simulink model "Control_Scheme_Joint_PID_Simulink"  (R2021a)
settings: Solver=FixedStepAuto  StartTime=0.0  StopTime=8  FixedStep=0.001  RelTol=1e-20
libraries: simulink x10, pid_lib x8
(part 2 of 2)

== matlab function Control_Scheme_Joint_PID_Simulink/MATLAB Function5 ==
  data: tao_in input; q output; t_in input; q_1 input; q_dot_1 input; q_dot output
function [q,q_dot] = SCDPR_Func(tao_in,t_in,q_1,q_dot_1)
% 主要求解电机的动力学方程，通过给定电机转矩以及索力信息，得到电机的角度以及角速度
%   此处显示详细说明

% global tao;
tao=tao_in;
% global tt;
tt=t_in;
% global Im;
Im=[0.1 0.1 0.1 0.1 0.1 0.1 0.1 0.1 0.1]';
% global Fv;
Fv=[1 1 1 1 1 1 1 1]';
% global Fs;
Fs=[1 1 1 1 1 1 1 1]';
% global R;
R=[0.0225 0.0225 0.0225 0.0225 0.0225 0.0225 0.0225 0.0225]';

T=0.001;
% T=0.01;

q=zeros(8,1);
q_dot=zeros(8,1);


% 第1个微分方程
Y11=q_1(1);
Y21=q_dot_1(1);
% 解微分方程
[t,q1] = ode45(@vdp1,[0 T],[Y11; Y21],[],tao,tt,Im,Fv,Fs,R);
q(1)=q1(end,1);
q_dot(1)=q1(end,2);

% 第2个微分方程
Y12=q_1(2);
Y22=q_dot_1(2);
% 解微分方程
[t,q2] = ode45(@vdp2,[0 T],[Y12; Y22],[],tao,tt,Im,Fv,Fs,R);
q(2)=q2(end,1);
q_dot(2)=q2(end,2);

% 第3个微分方程
Y13=q_1(3);
Y23=q_dot_1(3);
% 解微分方程
[t,q3] = ode45(@vdp3,[0 T],[Y13; Y23],[],tao,tt,Im,Fv,Fs,R);
q(3)=q3(end,1);
q_dot(3)=q3(end,2);

% 第4个微分方程
Y14=q_1(4);
Y24=q_dot_1(4);
% 解微分方程
[t,q4] = ode45(@vdp4,[0 T],[Y14; Y24],[],tao,tt,Im,Fv,Fs,R);
q(4)=q4(end,1);
q_dot(4)=q4(end,2);

% 第5个微分方程
Y15=q_1(5);
Y25=q_dot_1(5);
% 解微分方程
[t,q5] = ode45(@vdp5,[0 T],[Y15; Y25],[],tao,tt,Im,Fv,Fs,R);
q(5)=q5(end,1);
q_dot(5)=q5(end,2);

% 第6个微分方程
Y16=q_1(6);
Y26=q_dot_1(6);
% 解微分方程
[t,q6] = ode45(@vdp6,[0 T],[Y16; Y26],[],tao,tt,Im,Fv,Fs,R);
q(6)=q6(end,1);
q_dot(6)=q6(end,2);

% 第7个微分方程
Y17=q_1(7);
Y27=q_dot_1(7);
% 解微分方程
[t,q7] = ode45(@vdp7,[0 T],[Y17; Y27],[],tao,tt,Im,Fv,Fs,R);
q(7)=q7(end,1);
q_dot(7)=q7(end,2);

% 第8个微分方程
Y18=q_1(8);
Y28=q_dot_1(8);
% 解微分方程
[t,q8] = ode45(@vdp8,[0 T],[Y18; Y28],[],tao,tt,Im,Fv,Fs,R);
q(8)=q8(end,1);
q_dot(8)=q8(end,2);

function dydt1 = vdp1(t,y,tao,tt,Im,Fv,Fs,R)
%     global tao;
%     global tt;
%     global Im;
%     global Fv;
%     global Fs;
%     global R;
    
    tao1=tao(1);
    tt1=tt(1);
    Im1=Im(1);
    Fv1=Fv(1);
    Fs1=Fs(1);
    R1=R(1);

    p = y(1);
    dp = y(2);
% 	ddp = -Im_inv*Fv*dp-Im_inv*Fs*sign(dp)+Im_inv*tao-Im_inv*R*tt;
    ddp = -Fv1/Im1*dp-Fs1/Im1*sign(dp)+tao1/Im1-R1/Im1*tt1;
    dydt1 = [dp; ddp];
end

function dydt2 = vdp2(t,y,tao,tt,Im,Fv,Fs,R)
%     global tao;
%     global tt;
%     global Im;
%     global Fv;
%     global Fs;
%     global R;
    
    tao2=tao(2);
    tt2=tt(2);
    Im2=Im(2);
    Fv2=Fv(2);
    Fs2=Fs(2);
    R2=R(2);

    p = y(1);
    dp = y(2);
% 	ddp = -Im_inv*Fv*dp-Im_inv*Fs*sign(dp)+Im_inv*tao-Im_inv*R*tt;
    ddp = -Fv2/Im2*dp-Fs2/Im2*sign(dp)+tao2/Im2-R2/Im2*tt2;
    dydt2 = [dp; ddp];
end

function dydt3 = vdp3(t,y,tao,tt,Im,Fv,Fs,R)
%     global tao;
%     global tt;
%     global Im;
%     global Fv;
%     global Fs;
%     global R;
    
    tao3=tao(3);
    tt3=tt(3);
    Im3=Im(3);
    Fv3=Fv(3);
    Fs3=Fs(3);
    R3=R(3);

    p = y(1);
    dp = y(2);
% 	ddp = -Im_inv*Fv*dp-Im_inv*Fs*sign(dp)+Im_inv*tao-Im_inv*R*tt;
    ddp = -Fv3/Im3*dp-Fs3/Im3*sign(dp)+tao3/Im3-R3/Im3*tt3;
    dydt3 = [dp; ddp];
end

function dydt4 = vdp4(t,y,tao,tt,Im,Fv,Fs,R)
%     global tao;
%     global tt;
%     global Im;
%     global Fv;
%     global Fs;
%     global R;
    
    tao4=tao(4);
    tt4=tt(4);
    Im4=Im(4);
    Fv4=Fv(4);
    Fs4=Fs(4);
    R4=R(4);

    p = y(1);
    dp = y(2);
% 	ddp = -Im_inv*Fv*dp-Im_inv*Fs*sign(dp)+Im_inv*tao-Im_inv*R*tt;
    ddp = -Fv4/Im4*dp-Fs4/Im4*sign(dp)+tao4/Im4-R4/Im4*tt4;
    dydt4 = [dp; ddp];
end

function dydt5 = vdp5(t,y,tao,tt,Im,Fv,Fs,R)
%     global tao;
%     global tt;
%     global Im;
%     global Fv;
%     global Fs;
%     global R;
    
    tao5=tao(5);
    tt5=tt(5);
    Im5=Im(5);
    Fv5=Fv(5);
    Fs5=Fs(5);
    R5=R(5);

    p = y(1);
    dp = y(2);
% 	ddp = -Im_inv*Fv*dp-Im_inv*Fs*sign(dp)+Im_inv*tao-Im_inv*R*tt;
    ddp = -Fv5/Im5*dp-Fs5/Im5*sign(dp)+tao5/Im5-R5/Im5*tt5;
    dydt5 = [dp; ddp];
end

function dydt6 = vdp6(t,y,tao,tt,Im,Fv,Fs,R)
%     global tao;
%     global tt;
%     global Im;
%     global Fv;
%     global Fs;
%     global R;
    
    tao6=tao(6);
    tt6=tt(6);
    Im6=Im(6);
    Fv6=Fv(6);
    Fs6=Fs(6);
    R6=R(6);

    p = y(1);
    dp = y(2);
% 	ddp = -Im_inv*Fv*dp-Im_inv*Fs*sign(dp)+Im_inv*tao-Im_inv*R*tt;
    ddp = -Fv6/Im6*dp-Fs6/Im6*sign(dp)+tao6/Im6-R6/Im6*tt6;
    dydt6 = [dp; ddp];
end


function dydt7 = vdp7(t,y,tao,tt,Im,Fv,Fs,R)
%     global tao;
%     global tt;
%     global Im;
%     global Fv;
%     global Fs;
%     global R;
    
    tao7=tao(7);
    tt7=tt(7);
    Im7=Im(7);
    Fv7=Fv(7);
    Fs7=Fs(7);
    R7=R(7);

    p = y(1);
    dp = y(2);
% 	ddp = -Im_inv*Fv*dp-Im_inv*Fs*sign(dp)+Im_inv*tao-Im_inv*R*tt;
    ddp = -Fv7/Im7*dp-Fs7/Im7*sign(dp)+tao7/Im7-R7/Im7*tt7;
    dydt7 = [dp; ddp];
end

function dydt8 = vdp8(t,y,tao,tt,Im,Fv,Fs,R)
%     global tao;
%     global tt;
%     global Im;
%     global Fv;
%     global Fs;
%     global R;
    
    tao8=tao(8);
    tt8=tt(8);
    Im8=Im(8);
    Fv8=Fv(8);
    Fs8=Fs(8);
    R8=R(8);

    p = y(1);
    dp = y(2);
% 	ddp = -Im_inv*Fv*dp-Im_inv*Fs*sign(dp)+Im_inv*tao-Im_inv*R*tt;
    ddp = -Fv8/Im8*dp-Fs8/Im8*sign(dp)+tao8/Im8-R8/Im8*tt8;
    dydt8 = [dp; ddp];
end
end

== matlab function Control_Scheme_Joint_PID_Simulink/MATLAB Function6 ==
  data: t input; q_1 output size=[8,1] [8..8]; qd input; qd_dot input; q input; q_dot input; q_dot_1 output
function [q_1,q_dot_1] = Select_q_and_q_dot(t,qd,qd_dot,q,q_dot)

q_1=zeros(8,1);
q_dot_1=zeros(8,1);

if t<=3e-3
    q_1=qd;
    q_dot_1=qd_dot;
else
    q_1=q;
    q_dot_1=q_dot;
%     q_dot_1=qd_dot;
end

end

== matlab function Control_Scheme_Joint_PID_Simulink/MATLAB Function7 ==
  data: p input; t output; theta input; we input; bool output
function [t,bool] = Tension_Distribution_Func(p,theta,we)
% 求解索力分布的函数
% 输入：p 动平台位置 3*1
%      theta 动平台坐标系XYZ欧拉角 3*1
%      we 动平台受到的wrench 6*1(包含本身质量)
% 输出：t 绳索的张力的大小 8*1

g=9.81; %重力加速度
theta=theta';
x=theta(1);
y=theta(2);
z=theta(3);
Rxyz=Theta2RotationMatrix_Func(x,y,z);
f=we;
%% CoGiRo的参数 8绳索6自由度的CDPRs
% ai的定义
a1=[-7.5 -5.5 6]';
a2=[-7.5 -5.5 6]';
a3=[-7.5 5.5 6]';
a4=[-7.5 5.5 6]';
a5=[7.5 5.5 6]';
a6=[7.5 5.5 6]';
a7=[7.5 -5.5 6]';
a8=[7.5 -5.5 6]';
% bi的定义
b1=Rxyz*[0.5 -0.5 0]';
b2=Rxyz*[-0.5 0.5 1]';
b3=Rxyz*[-0.5 -0.5 0]';
b4=Rxyz*[0.5 0.5 1]';
b5=Rxyz*[-0.5 0.5 0]';
b6=Rxyz*[0.5 -0.5 1]';
b7=Rxyz*[0.5 0.5 0]';
b8=Rxyz*[-0.5 -0.5 1]';
% 绳索张力的上下限
tM=1000;
tm=10;
%% li=ai-bi-p,然后归一化li得到si=li/norm(li)
% li=ai-bi-p
l1=a1-b1-p;
l2=a2-b2-p;
l3=a3-b3-p;
l4=a4-b4-p;
l5=a5-b5-p;
l6=a6-b6-p;
l7=a7-b7-p;
l8=a8-b8-p;
% for i=1:8
%     expr=['l',num2str(i),'=a',num2str(i),'-b',num2str(i),'-p;'];
%     eval(expr);
% end
% si=li/norm(li)
s1=l1/norm(l1);
s2=l2/norm(l2);
s3=l3/norm(l3);
s4=l4/norm(l4);
s5=l5/norm(l5);
s6=l6/norm(l6);
s7=l7/norm(l7);
s8=l8/norm(l8);

% for i=1:8
%     expr=['s',num2str(i),'=l',num2str(i),'./norm(l',num2str(i),');'];
%     eval(expr);
% end

%% 构建W矩阵
% wi=[si;cross(bi,si)]
w1=[s1;cross(b1,s1)];
w2=[s2;cross(b2,s2)];
w3=[s3;cross(b3,s3)];
w4=[s4;cross(b4,s4)];
w5=[s5;cross(b5,s5)];
w6=[s6;cross(b6,s6)];
w7=[s7;cross(b7,s7)];
w8=[s8;cross(b8,s8)];
W=[w1 w2 w3 w4 w5 w6 w7 w8];

W_plus=pinv(W);
N=null(W);
tp=W_plus*f;

tm_vec=[tm;tm;tm;tm;tm;tm;tm;tm;];
tM_vec=[tM;tM;tM;tM;tM;tM;tM;tM;];

% line_select=[];
% langda_select=[];

find=0;
k_vector_all=[1;2;3;4;5;6;7;8];

%% 寻找第一个顶点vinit
i=1;
j=2;
bi=tm;
bj=tm;
bk_1=0;
bk_2=0;
ni=N(i,:);
nj=N(j,:);
tpi=tp(i,:);
tpj=tp(j,:);
A=[ni;nj];
b=[bi-tpi;bj-tpj];
langda=A\b; %2*1向量
vij=langda;

% line_select=[line_select;j];
% line_select=[line_select;i];
line_select=[i];

lk_1=i;
lk_2=j;

% line_find=[];
% line_find=[line_find;1];
% line_find=[line_find;2];
line_find=[i;j];

for i=3:8
    ni_2=N(i,:);
    tpi_2=tp(i,:);
    if ni_2*langda>=tm-tpi_2 & ni_2*langda<=tM-tpi_2
        line_find=[line_find;i];
    end
    
end

langda_select=[vij];


k_vector=setdiff(k_vector_all,line_select);

%% 循环找下一个节点，直到找到vk==vf
vk=[1e30;1e30];
% alpah_v=[1e30;1e30];
alpah_v=[1e30];
vk_1=vij;
nk_1=ni;
nk_2=nj;
nk_1_vertical=null(nk_1)';
nk_2_vertical=null(nk_2)';
l=0;
bk=0;
tpk=0;
count=0;
find2=0;
vf=vij;
vf_count=count+1;
nk_1_vertical_final=[0 0];
while(1)
%     alpah_k=[1e30;1e30];
    alpah_k=[1e30];
    count=count+1;
    find2=0;
    nk_1_vertical_final=[0 0];
    for i=1:length(k_vector)
        k=k_vector(i);
        nk=N(k,:);
        tpk=tp(k,:);
        
        % 考虑bj=tm情况
        if bk_2==0           
            nk_1_vertical_1=[nk_1(2) -nk_1(1)];
            nk_1_vertical_2=[-nk_1(2) nk_1(1)];
%             nk_1_vertical_1=[-nk_1(2) nk_1(1)];
%             nk_1_vertical_2=[nk_1(2) -nk_1(1)];
            if nk_2*nk_1_vertical_1'>=0
                nk_1_vertical=nk_1_vertical_1;
            else
                nk_1_vertical=nk_1_vertical_2;
            end           
            
            if nk*nk_1_vertical'>0
                if k==lk_2
                    if nk*vk_1<=tm-tpk
                        alpah_k=(tM-tpk-nk*vk_1)/(nk*nk_1_vertical');
                        bk_tmp=1;
                    elseif nk*vk_1>tm-tpk & nk*vk_1<=tM-tpk
                        alpah_k=(tM-tpk-nk*vk_1)/(nk*nk_1_vertical');
                        bk_tmp=1;
                    else
                        bk_tmp=0;
                    end
%                     if nk*vk_1>tm-tpk & nk*vk_1<=tM-tpk
%                         alpah_k=(tM-tpk-nk*vk_1)/(nk*nk_1_vertical');
%                         bk_tmp=1;
%                     end
                else
                    if nk*vk_1<=tm-tpk
                        alpah_k=(tm-tpk-nk*vk_1)/(nk*nk_1_vertical');
                        bk_tmp=0;
                    elseif nk*vk_1>tm-tpk & nk*vk_1<=tM-tpk
                        alpah_k=(tM-tpk-nk*vk_1)/(nk*nk_1_vertical');
                        bk_tmp=1;
                    else
                        bk_tmp=0;
                    end
%                     if nk*vk_1>tm-tpk & nk*vk_1<=tM-tpk
%                         alpah_k=(tM-tpk-nk*vk_1)/(nk*nk_1_vertical');
%                         bk_tmp=1;
%                     end
                end
                if (alpah_k<alpah_v) & alpah_k>=1e-6
                    alpah_v=alpah_k;
                    l=k;
                    find2=1;
                    nk_1_vertical_final=nk_1_vertical;
                    bk=bk_tmp;
                else
                    
                end
            end

            if nk*nk_1_vertical'<0
                if k==lk_2
                    if nk*vk_1>=tM-tpk
                        alpah_k=(tm-tpk-nk*vk_1)/(nk*nk_1_vertical');
                        bk_tmp=0;
                    elseif nk*vk_1>=tm-tpk & nk*vk_1<tM-tpk
                        alpah_k=(tm-tpk-nk*vk_1)/(nk*nk_1_vertical');
                        bk_tmp=0;
                    else
                        bk_tmp=0;
                    end
%                     if nk*vk_1>=tm-tpk & nk*vk_1<tM-tpk
%                         alpah_k=(tm-tpk-nk*vk_1)/(nk*nk_1_vertical');
%                         bk_tmp=0;
%                     end
                else
                    if nk*vk_1>=tM-tpk
                        alpah_k=(tM-tpk-nk*vk_1)/(nk*nk_1_vertical');
                        bk_tmp=1;
                    elseif nk*vk_1>=tm-tpk & nk*vk_1<tM-tpk
                        alpah_k=(tm-tpk-nk*vk_1)/(nk*nk_1_vertical');
                        bk_tmp=0;
                    else
                        bk_tmp=0;
                    end
%                     if nk*vk_1>=tm-tpk & nk*vk_1<tM-tpk
%                         alpah_k=(tm-tpk-nk*vk_1)/(nk*nk_1_vertical');
%                         bk_tmp=0;
%                     end
                end
                if (alpah_k<alpah_v) & alpah_k>=1e-6
                    alpah_v=alpah_k;
                    l=k;
                    find2=1;
                    nk_1_vertical_final=nk_1_vertical;
                    bk=bk_tmp;
                else
                    
                end
            end
        
        % 考虑bk=tM的情况
        elseif bk_2==1
            nk_1_vertical_1=[nk_1(2) -nk_1(1)];
            nk_1_vertical_2=[-nk_1(2) nk_1(1)];
%             nk_1_vertical_1=[-nk_1(2) nk_1(1)];
%             nk_1_vertical_2=[nk_1(2) -nk_1(1)];
            if nk_2*nk_1_vertical_1'<=0
                nk_1_vertical=nk_1_vertical_1;
            else
                nk_1_vertical=nk_1_vertical_2;
            end

            if nk*nk_1_vertical'>0
                if k==lk_2
                    if nk*vk_1<=tm-tpk
                        alpah_k=(tM-tpk-nk*vk_1)/(nk*nk_1_vertical');
                        bk_tmp=1;
                    elseif nk*vk_1>tm-tpk & nk*vk_1<=tM-tpk
                        alpah_k=(tM-tpk-nk*vk_1)/(nk*nk_1_vertical');
                        bk_tmp=1;
                    else
                        bk_tmp=0;
                    end
%                     if nk*vk_1>tm-tpk & nk*vk_1<=tM-tpk
%                         alpah_k=(tM-tpk-nk*vk_1)/(nk*nk_1_vertical');
%                         bk_tmp=1;
%                     end
                else
                    if nk*vk_1<=tm-tpk
                        alpah_k=(tm-tpk-nk*vk_1)/(nk*nk_1_vertical');
                        bk_tmp=0;
                    elseif nk*vk_1>tm-tpk & nk*vk_1<=tM-tpk
                        alpah_k=(tM-tpk-nk*vk_1)/(nk*nk_1_vertical');
                        bk_tmp=1;
                    else
                        bk_tmp=0;
                    end
%                     if nk*vk_1>tm-tpk & nk*vk_1<=tM-tpk
%                         alpah_k=(tM-tpk-nk*vk_1)/(nk*nk_1_vertical');
%                         bk_tmp=1;
%                     end
                end
                if (alpah_k<alpah_v) & alpah_k>=1e-6
                    alpah_v=alpah_k;
                    l=k;
                    find2=1;
                    nk_1_vertical_final=nk_1_vertical;
                    bk=bk_tmp;
                else
                    
                end
            end

            if nk*nk_1_vertical'<0
                if k==lk_2
                    if nk*vk_1>=tM-tpk
                        alpah_k=(tm-tpk-nk*vk_1)/(nk*nk_1_vertical');
                        bk_tmp=0;
                    elseif nk*vk_1>=tm-tpk & nk*vk_1<tM-tpk
                        alpah_k=(tm-tpk-nk*vk_1)/(nk*nk_1_vertical');
                        bk_tmp=0;
                    else
                        bk_tmp=0;
                    end
%                     if nk*vk_1>=tm-tpk & nk*vk_1<tM-tpk
%                         alpah_k=(tm-tpk-nk*vk_1)/(nk*nk_1_vertical');
%                         bk_tmp=0;
%                     end
                else
                    if nk*vk_1>=tM-tpk
                        alpah_k=(tM-tpk-nk*vk_1)/(nk*nk_1_vertical');
                        bk_tmp=1;
                    elseif nk*vk_1>=tm-tpk & nk*vk_1<tM-tpk
                        alpah_k=(tm-tpk-nk*vk_1)/(nk*nk_1_vertical');
                        bk_tmp=0;
                    else
                        bk_tmp=0;
                    end
%                     if nk*vk_1>=tm-tpk & nk*vk_1<tM-tpk
%                         alpah_k=(tm-tpk-nk*vk_1)/(nk*nk_1_vertical');
%                         bk_tmp=0;
%                     end
                end
                if (alpah_k<alpah_v) & alpah_k>=1e-6
                    alpah_v=alpah_k;
                    l=k;
                    find2=1;
                    nk_1_vertical_final=nk_1_vertical;
                    bk=bk_tmp;
                else
                    
                end
            end
        else
            find2=0;
        end
    end
    if find2==0 || count>1000
        t=[0 0 0 0 0 0 0 0]';
        bool=0;
%         disp("索力分布无解");
        break
    else
        vk=vk_1+alpah_v.*nk_1_vertical_final';
        nk=N(l,:);
        langda_select=[langda_select,vk];
    %     line_select(1,:)=line_select(2,:);
    %     line_select(2,:)=l;
        line_select(1)=l;
        lk=l;
        k_vector=setdiff(k_vector_all,line_select);
        vk_2=vk_1;
        vk_1=vk;
        nk_2=nk_1;
        nk_1=nk;
        bk_2=bk_1;
        bk_1=bk;
        lk_2=lk_1;
        lk_1=lk;
    %     alpah_v=[1e10;1e10];
        alpah_v=[1e30];

        if ~ismember(l,line_find)
            line_find=[line_find;l];
            line_find=sort(line_find);
            vf=vk;
            vf_count=count+1;
        else
            if abs(vf(1)-vk(1))<1e-3 & abs(vf(2)-vk(2))<1e-3
                line_find=sort(line_find);
                if isequal(line_find,k_vector_all)
%                     disp('查找成功');
                    bool=1;
                    break;
                else
                    t=[0 0 0 0 0 0 0 0]';
                    bool=0;
%                     disp('查找失败');
                    return
                end
            else
                line_find=line_find;
            end
        end        
    end
    
end

langda_final_vce=langda_select(1:2,end-(size(langda_select,2)-vf_count):end-1);

%% 重心法得到多边形质心
% 求解A
A=0;
vc1=0;
vc2=0;

count=size(langda_select,2)-vf_count;

if count==3
    vc1=(langda_final_vce(1,1)+langda_final_vce(1,2)+langda_final_vce(1,3))/3;
    vc2=(langda_final_vce(2,1)+langda_final_vce(2,2)+langda_final_vce(2,3))/3;
end

if count==4
    vc1=(langda_final_vce(1,1)+langda_final_vce(1,2)+langda_final_vce(1,3)+langda_final_vce(1,4))/4;
    vc2=(langda_final_vce(2,1)+langda_final_vce(2,2)+langda_final_vce(2,3)+langda_final_vce(2,4))/4;
end

if count>4
    for p=1:size(langda_final_vce,2)-1
        A=A+(langda_final_vce(1,p)*langda_final_vce(2,p+1)-langda_final_vce(1,p+1)*langda_final_vce(2,p))/2;
    end

    for p=1:size(langda_final_vce,2)-1
        vc1=vc1+((langda_final_vce(1,p)+langda_final_vce(1,p+1))*(langda_final_vce(1,p)*langda_final_vce(2,p+1)-langda_final_vce(1,p+1)*langda_final_vce(2,p)))/(6*A);
        vc2=vc2+((langda_final_vce(2,p)+langda_final_vce(2,p+1))*(langda_final_vce(1,p)*langda_final_vce(2,p+1)-langda_final_vce(1,p+1)*langda_final_vce(2,p)))/(6*A);
    end
end

% vc1=456.6389;
% vc2=534.3178;

langda_final=[vc1 vc2]';
t=tp+N*langda_final;

end

== matlab function Control_Scheme_Joint_PID_Simulink/MATLAB Function8 ==
  data: q input; p output; theta output
function [p,theta] = ForwardKenamatics_Func(q)
%*********************************************************
%使用LM法求解运动学正解，迭代起点在base内部空间任意选择；
%输入参数：L 绳索长度构成的行向量；
%输出参数：solution 动平台的位姿向量
%         k 迭代次数
%         minF 误差F的最终值
%*********************************************************
%%
%base/plateform的基本数据：
%base:L*W*H=15*11*6
%drawing points在O-XYZ中表示：

A=zeros(3,8);
Bp=zeros(3,8);

A(1:3,1)=[-7.5 -5.5 6]';
A(1:3,2)=[-7.5 -5.5 6];
A(1:3,3)=[-7.5 5.5 6]';
A(1:3,4)=[-7.5 5.5 6]';
A(1:3,5)=[7.5 5.5 6]';
A(1:3,6)=[7.5 5.5 6];
A(1:3,7)=[7.5 -5.5 6];
A(1:3,8)=[7.5 -5.5 6]';
%plateform:l*w*h=1*1*1
%attach points在P-XpYpZp中表示：
Bp(1:3,1)=[0.5 -0.5 0]';
Bp(1:3,2)=[-0.5 0.5 1]';
Bp(1:3,3)=[-0.5 -0.5 0]';
Bp(1:3,4)=[0.5 0.5 1]';
Bp(1:3,5)=[-0.5 0.5 0]';
Bp(1:3,6)=[0.5 -0.5 1]';
Bp(1:3,7)=[0.5 0.5 0]';
Bp(1:3,8)=[-0.5 -0.5 1]';

%%
%约束函数向量为vector_f；目标函数为F;
%采用《methods for non-linear least squares problems》中表述：F=1/2*sum(fi(x)^2)=1/2*(vector_f'*vector_f)
l=0.0225*q';
length_given=l;
%下面为LM法参数：
%设置stop criteria:
epsilon1=1.0e-8;
epsilon2=1.0e-8;
%设置迭代次数上限：
k_max=100;
%当前迭代次数：
k=0;
%设置初始迭代位置:设置为固定平台中心位置
%pose_position_angle=[x y z angle_x angle_y angle_z]
pose_position_angle=[0 0 1 0 0 0];
%u的增长因子v
v=2;
%结束标志
found=false;

%% 统计时间的开始
%LM算法计算开始：
jacobian_f=Jaco(pose_position_angle,A,Bp);
A_matrix=jacobian_f'*jacobian_f;
vector_f=FunctionVector_f(pose_position_angle,A,Bp,length_given);
g=jacobian_f'*vector_f;

if norm(g)<=epsilon1
    found=true;
end

%设置初始damped parameter u
tau=1.0e-3;
u=tau*max([A_matrix(1,1),A_matrix(2,2),A_matrix(3,3),A_matrix(4,4),A_matrix(5,5),A_matrix(6,6)]);

while(found==false)&&(k<=k_max)
    k=k+1;
    %解的迭代方向及步长
    h_lm=(A_matrix+u*eye(6,6))\(-1*g);
    %h_lm=inv(A_matrix+u*eye(6,6))*(-1*g);
    if norm(h_lm)<=(epsilon2*(norm(pose_position_angle))+epsilon2)
        found=true;
    else
        pose_position_angle_new=pose_position_angle+h_lm';
        vector_f_new=FunctionVector_f(pose_position_angle_new,A,Bp,length_given);
        %计算更新指标Q
        Q=Q_criteria(vector_f,vector_f_new,h_lm,u,g);
        
        if Q>0
            
            pose_position_angle=pose_position_angle_new;
            
            jacobian_f=Jaco(pose_position_angle,A,Bp);
            A_matrix=jacobian_f'*jacobian_f;
            vector_f=FunctionVector_f(pose_position_angle,A,Bp,length_given);
            g=jacobian_f'*vector_f;
            
            if norm(g)<=epsilon1
                found=true;
            end
            u=u*max([1/3, 1, 1-(2*Q-1)^3]);
            v=2;
        else
            u=u*v;
            v=2*v;
        end
        
    end
    
    
end

solution=pose_position_angle';
p=solution(1:3,1);
theta=solution(4:6,1)/pi*(180);

end
